simulink model "CanonicalMax2"  (R2020a)
settings: Solver=VariableStepAuto  StartTime=0.0  StopTime=20  RelTol=1e-3
settings Model: Creator=Lenovo  LastModifiedBy=Lenovo

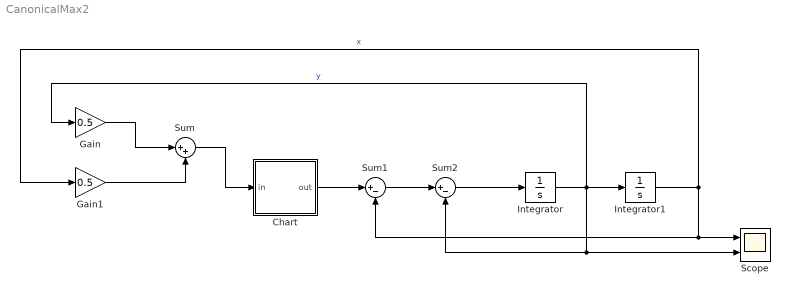
== system CanonicalMax2 ==
  Chart : Stateflow chart  TreatAsAtomicUnit=on
  Gain : Gain  Gain=0.5
  Gain1 : Gain  Gain=0.5
  Integrator : Integrator  InitialCondition=1
  Integrator1 : Integrator  InitialCondition=1
  Scope : Scope  NumInputPorts=2
  Sum : Sum  Inputs=|++
  Sum1 : Sum  Inputs=|+-
  Sum2 : Sum  Inputs=|+-
  wires:
  Gain/1 -> Sum/1
  Gain1/1 -> Sum/2
  Sum1/1 -> Sum2/1
  Sum2/1 -> Integrator/1
  Integrator/1 -> Gain/1, Scope/2, Sum2/2, Integrator1/1  "y"
  Integrator1/1 -> Sum1/2, Scope/1, Gain1/1  "x"
  Sum/1 -> Chart/1(in)
  Chart/1(out) -> Sum1/1

== stateflow chart CanonicalMax2/Chart ==
  settings: updateMethod=DISCRETE  sampleTime=1
  state A
    du: out = in;
  state B
    du: out = 0;
  (default) -> A
  B -> A : [in > 0]
  A -> B : [in < 0]
  data: in input; out output
